simulink model "IsometricContractions"  (R2012b)
settings: Solver=ode1  StartTime=0.0  StopTime=7  FixedStep=0.001  RelTol=1e-3
undefined symbols (not defined in the file): HIL, LCconv, sat, thresh
libraries: quarc_library x4, ScienceStimHasomed_Lib x1, simulink x1
settings Model: SimulationMode=external  ExtModeTrigDuration=5000000  Creator=LabUser  LastModifiedBy=LabUser
settings SolverCC: PositivePriorityOrder=on
settings DataIOCC: LimitDataPoints=off
settings DebuggingCC: SolverPrmCheckMsg=none
settings RTWCC: SystemTargetFile=quarc_win64.tlc  TemplateMakefile=quarc_default_tmf  Description=QUARC Win64 Target  ProcessScript=quarc_win64_make_rtw_hook
settings RTWCC: CustomLibrary=|
  | sciencemode.obj
  | serial_windows.obj
settings STFCustomTargetCC: TargetPreCompLibLocation=C:\PROGRA~3\QUARC\lib\2012b\win64\release  CodeReplacementLibrary=ANSI_C  GeneratePreprocessorConditionals=Disable all  CombineOutputUpdateFcns=on  GRTInterface=off  SystemTargetFile=quarc_win64.tlc
settings GRTTargetCC: TargetPreCompLibLocation=C:\PROGRA~3\QUARC\lib\2012b\win64\release  ParMdlRefBuildCompliant=off  CompOptLevelCompliant=off  ConcurrentExecutionCompliant=off  MatFileLogging=off  ExtMode=on  ExtModeMexFile=quarc_comm

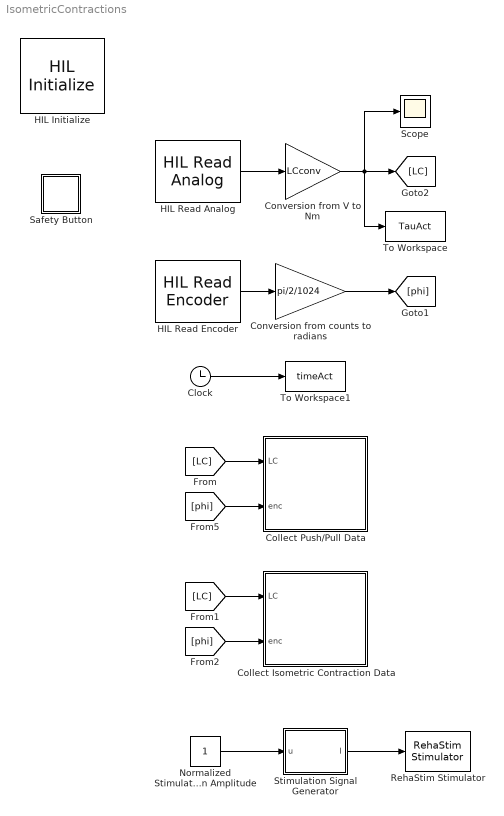
== system IsometricContractions ==
  Clock : Clock
  Collect Isometric Contraction Data : Subsystem
  Collect Push/Pull Data : Subsystem
  Conversion from V to Nm : Gain  Gain=LCconv
  Conversion from counts to radians : Gain  Gain=pi/2/1024
  HIL Initialize : quarc_library/Data Acquisition/Generic/Configuration/HIL Initialize  Priority=-99  object_name=HIL-1  board_type=qpid_e  board_number=0  board_options=enc0_dir=0;enc0_filter=1;enc0_a=1;enc0_b=1;enc0_z=0;enc0_reload=0;enc1_dir=0;enc1_filter=1;enc1_a=1;enc1_b=1;enc1_z=0;enc1_reload=0;enc2_dir=0;enc2_filter=1;enc2_a=1;enc2_b=1;enc2_z=0;enc2_reload=0;enc3_dir=0;enc3_filter=1;enc3_a=1;enc3_b=1;enc3_z=0;enc3_reload=0;enc4_dir=0;enc4_filter=1;enc4_a=1;enc4_b=1;enc4_z=0;enc4_reload=0;enc5_dir=0;enc5_filter=1;enc5_a=1;enc5_b=1;enc5_z=0;enc5_reload=0;enc6_dir=0;enc6_filter=1;enc6_a=1;enc6_b=1;enc6_z=0;enc6_reload=0;enc7_dir=0;enc7_filter=1;enc7_a=1;enc7_b=1;enc7_z=0;enc7_reload=0;ext_int_polarity=0;fuse_polarity=0;convert_polarity=0;watchdog_polarity=0;ext_int_watchdog=0;fuse_watchdog=0;trig1_watchdog=0;watchdog_to_trig1=0;watchdog_to_trig2=0;counter_to_trig0=0;trigger_adcs=0;latch_on_adc=0;pwm_immediate=0  exclusive=off  active=off  hardware_clocks=[0:16]  clock_modes=[]  initial_clock_frequencies=[]  set_clock_params_at_start=off  set_clock_params_at_switch_in=off  set_clock_frequencies_at_start=off  set_clock_frequencies_at_switch_in=off  analog_input_channels=[0:7]  analog_input_maximums=10  analog_input_minimums=-10  set_analog_input_params_at_start=off  set_analog_input_params_at_switch_in=off  analog_output_channels=[0:7]  analog_output_maximums=10  analog_output_minimums=-10  initial_analog_outputs=[0]  final_analog_outputs=[0]  watchdog_analog_outputs=0  set_analog_output_params_at_start=off  set_analog_output_params_at_switch_in=off  set_analog_outputs_at_start=on  set_analog_outputs_at_switch_in=off  set_analog_outputs_at_terminate=on  set_analog_outputs_at_switch_out=off  set_analog_outputs_on_watchdog=off  digital_input_channels=[]  digital_output_channels=[]  digital_output_configuration=[]  initial_digital_outputs=[1]  final_digital_outputs=[1]  watchdog_digital_outputs=[2]  set_digital_output_params_at_start=off  set_digital_output_params_at_switch_in=off  set_digital_outputs_at_start=on  set_digital_outputs_at_switch_in=off  set_digital_outputs_at_terminate=on  set_digital_outputs_at_switch_out=off  set_digital_outputs_on_watchdog=off  encoder_channels=[0:7]  quadrature=[4]  encoder_filter_frequency=40e6/1  initial_encoder_counts=[0]  set_encoder_params_at_start=on  set_encoder_params_at_switch_in=off  set_encoder_counts_at_start=off  set_encoder_counts_at_switch_in=off  pwm_channels=[0:7]  pwm_modes=0  pwm_frequency=40e6/4096  pwm_configuration=[0]  pwm_alignment=[0]  pwm_polarity=[1]  pwm_leading_deadband=[0]  pwm_trailing_deadband=[0]  initial_pwm_outputs=[0]  final_pwm_outputs=[0]  watchdog_pwm_outputs=[0]  set_pwm_params_at_start=on  set_pwm_params_at_switch_in=off  set_pwm_outputs_at_start=on  set_pwm_outputs_at_switch_in=off  set_pwm_outputs_at_terminate=on  set_pwm_outputs_at_switch_out=off  set_pwm_outputs_on_watchdog=off  other_output_channels=[]  initial_other_outputs=[]  final_other_outputs=[]  watchdog_other_outputs=[]  set_other_outputs_at_start=off  set_other_outputs_at_switch_in=off  set_other_outputs_at_terminate=off  set_other_outputs_at_switch_out=off  set_other_outputs_on_watchdog=off
  HIL Read Analog : quarc_library/Data Acquisition/Generic/Immediate I//O/HIL Read Analog  object_name=HIL-1  channels=0  sample_time=qc_get_step_size  active=on  vector_output=off
  HIL Read Encoder : quarc_library/Data Acquisition/Generic/Immediate I//O/HIL Read Encoder  object_name=HIL-1  channels=0  sample_time=qc_get_step_size  active=on  vector_output=off  data_type_mode=Inherit via back propagation  data_type=double
  Normalized Stimulation Amplitude : Constant
  RehaStim Stimulator : ScienceStimHasomed_Lib/RehaStim Stimulator  sFreq=1000  Freq=stimfreq  PWidth=PW
  Safety Button : Subsystem
  Scope : Scope
      settings: TimeRange=7  YMin=-25  YMax=250  MaxDataPoints=20001
  Stimulation Signal Generator : Subsystem
  To Workspace : ToWorkspace  VariableName=TauAct  SampleTime=-1
  To Workspace1 : ToWorkspace  VariableName=timeAct  SampleTime=-1
  wires:
  HIL Read Encoder/1 -> Conversion from counts to radians/1
  Conversion from counts to radians/1 -> [phi]
  [phi] -> Collect Push/Pull Data/2(enc)
  [LC] -> Collect Push/Pull Data/1(LC)
  [phi] -> Collect Isometric Contraction Data/2(enc)
  [LC] -> Collect Isometric Contraction Data/1(LC)
  HIL Read Analog/1 -> Conversion from V to Nm/1
  Conversion from V to Nm/1 -> Scope/1, To Workspace/1, [LC]
  Clock/1 -> To Workspace1/1
  Normalized Stimulation Amplitude/1 -> Stimulation Signal Generator/1(u)
  Stimulation Signal Generator/1(I) -> RehaStim Stimulator/1

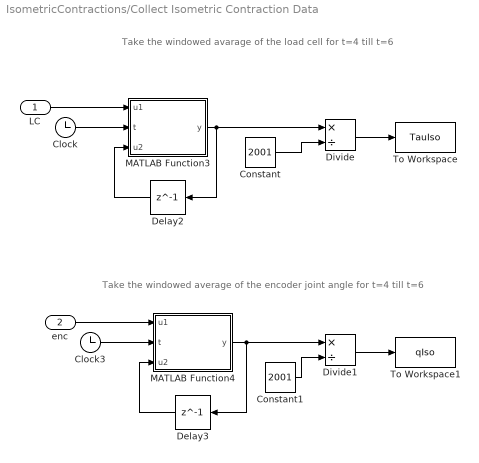
== system IsometricContractions/Collect Isometric Contraction Data ==
  note: Take the windowed avarage of the load cell for t=4 till t=6
  note: Take the windowed average of the encoder joint angle for t=4 till t=6
  LC : Inport
  enc : Inport  Port=2
  Clock : Clock
  Clock3 : Clock
  Constant : Constant  Value=2001
  Constant1 : Constant  Value=2001
  Delay2 : Delay  DelayLength=1  InitialCondition=0
  Delay3 : Delay  DelayLength=1  InitialCondition=0
  Divide : Product  Inputs=*/
  Divide1 : Product  Inputs=*/
  MATLAB Function3 : MATLAB Function  TreatAsAtomicUnit=on
  MATLAB Function4 : MATLAB Function  TreatAsAtomicUnit=on
  To Workspace : ToWorkspace  VariableName=TauIso  SampleTime=-1
      settings: MaxDataPoints=1
  To Workspace1 : ToWorkspace  VariableName=qIso  SampleTime=-1
      settings: MaxDataPoints=1
  wires:
  MATLAB Function3/1(y) -> Divide/1, Delay2/1
  Constant/1 -> Divide/2
  MATLAB Function4/1(y) -> Delay3/1, Divide1/1
  Constant1/1 -> Divide1/2
  Clock/1 -> MATLAB Function3/2(t)
  LC/1 -> MATLAB Function3/1(u1)
  Delay2/1 -> MATLAB Function3/3(u2)
  Clock3/1 -> MATLAB Function4/2(t)
  enc/1 -> MATLAB Function4/1(u1)
  Delay3/1 -> MATLAB Function4/3(u2)
  Divide/1 -> To Workspace/1
  Divide1/1 -> To Workspace1/1

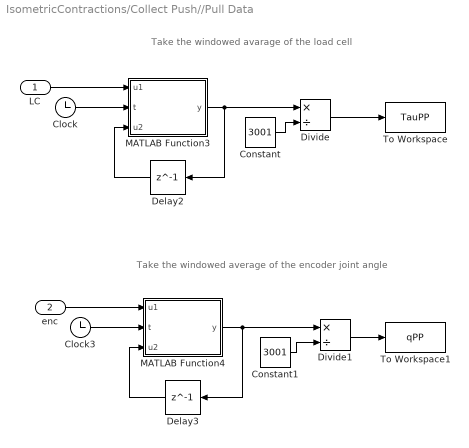
== system IsometricContractions/Collect Push//Pull Data ==
  note: Take the windowed avarage of the load cell
  note: Take the windowed average of the encoder joint angle
  LC : Inport
  enc : Inport  Port=2
  Clock : Clock
  Clock3 : Clock
  Constant : Constant  Value=3001
  Constant1 : Constant  Value=3001
  Delay2 : Delay  DelayLength=1  InitialCondition=0
  Delay3 : Delay  DelayLength=1  InitialCondition=0
  Divide : Product  Inputs=*/
  Divide1 : Product  Inputs=*/
  MATLAB Function3 : MATLAB Function  TreatAsAtomicUnit=on
  MATLAB Function4 : MATLAB Function  TreatAsAtomicUnit=on
  To Workspace : ToWorkspace  VariableName=TauPP  SampleTime=-1
      settings: MaxDataPoints=1
  To Workspace1 : ToWorkspace  VariableName=qPP  SampleTime=-1
      settings: MaxDataPoints=1
  wires:
  MATLAB Function3/1(y) -> Divide/1, Delay2/1
  Constant/1 -> Divide/2
  MATLAB Function4/1(y) -> Delay3/1, Divide1/1
  Constant1/1 -> Divide1/2
  Clock/1 -> MATLAB Function3/2(t)
  LC/1 -> MATLAB Function3/1(u1)
  Delay2/1 -> MATLAB Function3/3(u2)
  Clock3/1 -> MATLAB Function4/2(t)
  enc/1 -> MATLAB Function4/1(u1)
  Delay3/1 -> MATLAB Function4/3(u2)
  Divide/1 -> To Workspace/1
  Divide1/1 -> To Workspace1/1

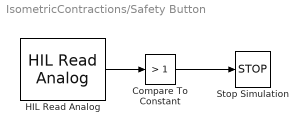
== system IsometricContractions/Safety Button ==
  Compare To Constant : simulink/Logic and Bit Operations/Compare To Constant  relop=>  const=1  OutDataTypeStr=boolean
  HIL Read Analog : quarc_library/Data Acquisition/Generic/Immediate I//O/HIL Read Analog  object_name=HIL-1  channels=[7]  sample_time=qc_get_step_size  active=on  vector_output=off
  Stop Simulation : Stop
  wires:
  HIL Read Analog/1 -> Compare To Constant/1
  Compare To Constant/1 -> Stop Simulation/1

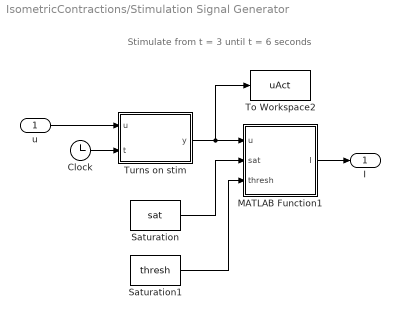
== system IsometricContractions/Stimulation Signal Generator ==
  note: Stimulate from t = 3 until t = 6 seconds
  u : Inport
  Clock : Clock
  MATLAB Function1 : MATLAB Function  TreatAsAtomicUnit=on
  Saturation : Constant  Value=sat
  Saturation1 : Constant  Value=thresh
  To Workspace2 : ToWorkspace  VariableName=uAct  SampleTime=-1
  Turns on stim : MATLAB Function  TreatAsAtomicUnit=on
  I : Outport
  wires:
  u/1 -> Turns on stim/1(u)
  Clock/1 -> Turns on stim/2(t)
  Turns on stim/1(y) -> To Workspace2/1, MATLAB Function1/1(u)
  MATLAB Function1/1(I) -> I/1
  Saturation/1 -> MATLAB Function1/2(sat)
  Saturation1/1 -> MATLAB Function1/3(thresh)

== matlab function IsometricContractions/Stimulation Signal Generator/MATLAB Function1 ==
  data: u input; I output; sat input; thresh input
function I = fcn(u,sat,thresh)

if u <= 0
    I = 0;
elseif u >= 1
    I = sat;
else
    I = thresh + u*(sat-thresh);
end

== matlab function IsometricContractions/Collect Isometric Contraction Data/MATLAB Function3 ==
  data: u1 input; y output; t input; u2 input
function y = fcn(u1,t,u2)

if (t >= 4) && (t <= 6)
    y = u1+u2;
else
    y = u2;
end

== matlab function IsometricContractions/Collect Isometric Contraction Data/MATLAB Function4 ==
  data: u1 input; y output; t input; u2 input
function y = fcn(u1,t,u2)

if (t >= 4) && (t <= 6)
    y = u1+u2;
else
    y = u2;
end

== matlab function IsometricContractions/Stimulation Signal Generator/Turns on stim ==
  data: u input; y output; t input
function y = fcn(u,t)

if (t >= 3) && (t <= 6)
    y = u;
else
    y = 0;
end

== matlab function IsometricContractions/Collect Push//Pull Data/MATLAB Function3 ==
  data: u1 input; y output; t input; u2 input
function y = fcn(u1,t,u2)

if t <= 3
    y = u1+u2;
else
    y = u2;
end

== matlab function IsometricContractions/Collect Push//Pull Data/MATLAB Function4 ==
  data: u1 input; y output; t input; u2 input
function y = fcn(u1,t,u2)

if t <= 3
    y = u1+u2;
else
    y = u2;
end
